simulink model "LQR_simulink_Sily_2024a"  (R2024a)
settings: Solver=FixedStepAuto  StartTime=0.0  StopTime=30  FixedStep=0.05  RelTol=1e-3
values from neighbouring files (symbols this model uses):
  Ac = LinSystem.Ac    [LQR_matlab_client_Otacky.m]    (also in LQR_matlab_client_Sily.m; LQR_sync_matlab_client.m; sync_matlab_client.m)
  b_moment = 5.4e-6    (= 5.4e-06)    [LQR_matlab_client_Otacky.m]    (also in LQR_matlab_client_Sily.m; LQR_sync_matlab_client.m; sync_matlab_client.m)
  Bc = LinSystem.Bc    [LQR_matlab_client_Otacky.m]    (also in LQR_matlab_client_Sily.m; LQR_sync_matlab_client.m; sync_matlab_client.m)
  Cc = LinSystem.Cc    [LQR_matlab_client_Otacky.m]    (also in LQR_matlab_client_Sily.m; LQR_sync_matlab_client.m; sync_matlab_client.m)
  Dc = LinSystem.Dc    [LQR_matlab_client_Otacky.m]    (also in LQR_matlab_client_Sily.m; LQR_sync_matlab_client.m; sync_matlab_client.m)
  k_thrust = 2.3e-3    (= 0.0023)    [LQR_matlab_client_Otacky.m]    (also in LQR_matlab_client_Sily.m; LQR_sync_matlab_client.m; sync_matlab_client.m)
  ki_lqr = K_ex_lqr(:, 17:20)    [LQR_koeficienty.m]
  kp_lqr = K_ex_lqr(:, 1:16)    [LQR_koeficienty.m]
  l = 0.2051    [LQR_matlab_client_Otacky.m]    (also in LQR_matlab_client_Sily.m; LQR_sync_matlab_client.m; sync_matlab_client.m)
  Q = 1e-3    (= 0.001)    [LQR_matlab_client_Otacky.m]    (also in LQR_matlab_client_Sily.m; LQR_sync_matlab_client.m; sync_matlab_client.m)
  R = 1e-4    (= 0.0001)    [LQR_matlab_client_Otacky.m]    (also in LQR_matlab_client_Sily.m; LQR_sync_matlab_client.m; sync_matlab_client.m)
  timestep = timeData.TimeStep    [LQR_matlab_client_Otacky.m]    (also in LQR_matlab_client_Sily.m; LQR_sync_matlab_client.m; sync_matlab_client.m)
  Us_p = [(M+m)*g; 0; 0; 0]    [LQR_matlab_client_Sily.m]    (also in LQR_sync_matlab_client.m)
  Xs_p = [0;0;0; 0;0;0; 0;0; 0;0;0; 0;0;0; 0;0]    [LQR_matlab_client_Otacky.m]    (also in LQR_matlab_client_Sily.m; LQR_sync_matlab_client.m)
undefined symbols (not defined in the file or in its folder): Continuous, Time
libraries: simulink_extras x5, simulink x1, ctrlSharedLib x1
settings Model: Creator=yaozhong.zhang  LastModifiedBy=Admin
settings DebuggingCC: UnconnectedInputMsg=warning  UnconnectedOutputMsg=warning  UnconnectedLineMsg=warning
settings ModelReferenceCC: EnableRefExpFcnMdlSchedulingChecks=on
settings RTWCC: GPUComputeCapability=3.5

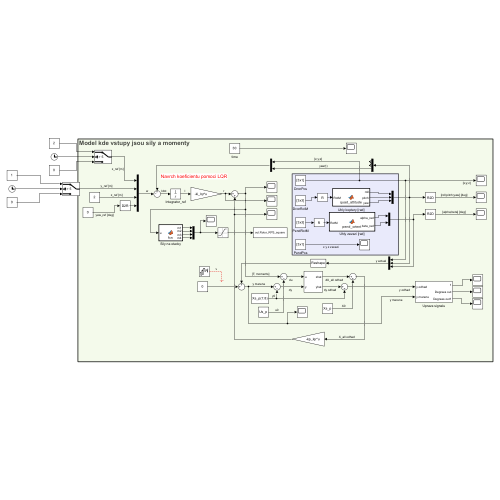
[thumbnail: Simulink's stored preview of the top-level diagram]
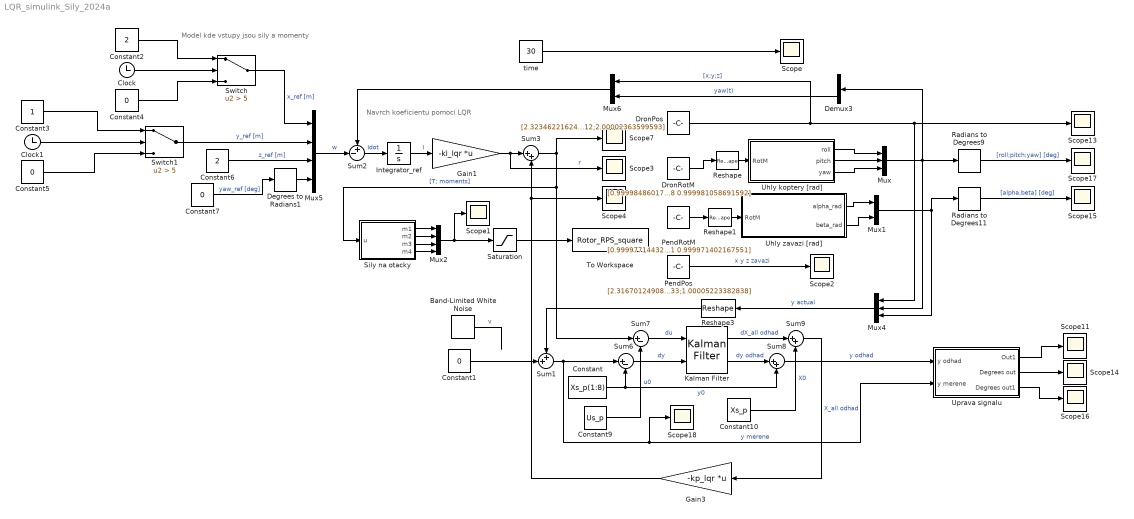
== system LQR_simulink_Sily_2024a ==
  note: Model kde vstupy jsou sily a momenty
  note: Navrch koeficientu pomoci LQR
  Band-Limited White Noise : simulink/Sources/Band-Limited White Noise  Cov=R*str2num(timestep)  Ts=str2num(timestep)  seed=[23341]
  Clock : Clock
  Clock1 : Clock
  Constant : Constant  Value=Xs_p(1:8)
  Constant{1,4..5,7} (4 alike) : Constant  Value=0
  Constant10 : Constant  Value=Xs_p
  Constant2 : Constant  Value=2
  Constant3 : Constant
  Constant6 : Constant  Value=2
  Constant9 : Constant  Value=Us_p
  Degrees to Radians1 : simulink_extras/Transformations/Degrees to Radians
  Demux3 : Demux  Outputs=3
  DronPos : Constant  Value=[2.32346221624764;1.16170882076612;2.00002363599593]  SampleTime=-1
  DronRotM : Constant  Value=[0.999984860177813 -5.50289297469162e-05 0.00550239829327193;3.98544005691727e-05 0.999996196263047 0.00275787437439109;-0.00550252912647141 -0.00275761332587778 0.999981058691592]  SampleTime=-1
  Gain1 : Gain  Gain=-ki_lqr  Multiplication=Matrix(K*u)
  Gain3 : Gain  Gain=-kp_lqr  Multiplication=Matrix(K*u)
  Integrator_ref : Integrator  InitialCondition=[1.74013379756829e-14;-1.44199272323054e-13;-17.1813439246218;-1.04137858173955e-14]
  Kalman Filter : ctrlSharedLib/Kalman Filter  TimeDomain=Continuous-Time  UseCurrentEstimator=on  ModelSource=Individual A, B, C, D matrices  ModelSourceVariable=ss(0.95,1,1,0,1)  A=Ac  B=Bc  C=Cc  D=Dc  NumberOfStates=1  NumberOfInputs=1  NumberOfOutputs=1  InitialEstimateSource=Dialog  X0=[0;0;2; 0;0;0; 0;0; 0;0;0; 0;0;0; 0;0]  P0=10  UseK=off  UseGH=off  NumberOfProcessNoiseInputs=1  G=1  TimeInvariantG=on  H=0  TimeInvariantH=on  Q=diag(Q*ones(16,1))  TimeInvariantQ=on  R=diag(R*ones(8,1))  TimeInvariantR=on  N=0  TimeInvariantN=on  AddInputPort=on  AddEnablePort=off  OutputEstimatedY=on  OutputP=off  Ts=-1
  Mux : Mux  Inputs=3
  Mux1 : Mux  Inputs=2
  Mux2 : Mux
  Mux4 : Mux  Inputs=3
  Mux5 : Mux
  Mux6 : Mux  Inputs=2
  PendPos : Constant  Value=[2.31670124908824;1.15831999056533;1.00005223382838]  SampleTime=-1
  PendRotM : Constant  Value=[0.999977144321402 -1.25651106658396e-05 0.00676096715939648;-1.03469676683034e-05 0.999994257844918 0.0033888302007973;-0.00676097091790106 -0.00338882270229201 0.999971402167551]  SampleTime=-1
  Radians to Degrees11 : simulink_extras/Transformations/Radians to Degrees
  Radians to Degrees9 : simulink_extras/Transformations/Radians to Degrees
  Reshape : Reshape  OutputDimensionality=Customize  OutputDimensions=[3,3]
  Reshape1 : Reshape  OutputDimensionality=Customize  OutputDimensions=[3,3]
  Reshape3 : Reshape  OutputDimensionality=Customize  OutputDimensions=[8,1]
  Saturation : Saturate  UpperLimit=4200  LowerLimit=0
  Scope{,1..4,7,11,13..18} (13 alike) : Scope
  Sily na otacky : MATLAB Function  TreatAsAtomicUnit=on
  Sum1 : Sum  Inputs=++|
  Sum2 : Sum  Inputs=+-|
  Sum3 : Sum  Inputs=|++
  Sum6 : Sum  Inputs=|+-
  Sum7 : Sum  Inputs=|+-
  Sum8 : Sum  Inputs=|++
  Sum9 : Sum  Inputs=|++
  Switch : Switch  Criteria=u2 > Threshold  Threshold=5  SaturateOnIntegerOverflow=off  InputSameDT=off
  Switch1 : Switch  Criteria=u2 > Threshold  Threshold=5  SaturateOnIntegerOverflow=off  InputSameDT=off
  To Workspace : ToWorkspace  VariableName=Rotor_RPS_square  SampleTime=-1
  Uhly koptery [rad] : MATLAB Function  TreatAsAtomicUnit=on
  Uhly zavazi [rad] : MATLAB Function  TreatAsAtomicUnit=on
  Uprava signalu : Subsystem
  time : Constant  Value=30  SampleTime=-1
  wires:
  DronRotM/1 -> Reshape/1
  Uhly koptery [rad]/2(pitch) -> Mux/2
  Uhly koptery [rad]/1(roll) -> Mux/1
  Uhly koptery [rad]/3(yaw) -> Mux/3
  PendPos/1 -> Scope2/1  "x y z zavazi"
  Reshape/1 -> Uhly koptery [rad]/1(RotM)
  PendRotM/1 -> Reshape1/1
  Reshape1/1 -> Uhly zavazi [rad]/1(RotM)
  Uhly zavazi [rad]/1(alpha_rad) -> Mux1/1
  Uhly zavazi [rad]/2(beta_rad) -> Mux1/2
  time/1 -> Scope/1
  Mux6/1 -> Sum2/1
  Gain3/1 -> Scope4/1, Sum3/2
  Sum2/1 -> Integrator_ref/1  "Idot"
  Switch1/1 -> Mux5/2  "y_ref [m]"
  Constant6/1 -> Mux5/3  "z_ref [m]"
  Uprava signalu/1(Out1) -> Scope11/1
  Radians to Degrees11/1 -> Scope15/1  "[alpha;beta] [deg]"
  Mux/1 -> Demux3/1, Radians to Degrees9/1, Mux4/2
  Mux4/1 -> Reshape3/1  "y actual"
  Uprava signalu/3(Degrees out1) -> Scope16/1
  Switch/1 -> Mux5/1  "x_ref [m]"
  Integrator_ref/1 -> Gain1/1  "I"
  Demux3/3 -> Mux6/2  "yaw(t)"
  Uprava signalu/2(Degrees out) -> Scope14/1
  Degrees to Radians1/1 -> Mux5/4
  Constant7/1 -> Degrees to Radians1/1  "yaw_ref [deg]"
  DronPos/1 -> Scope13/1, Mux4/1, Mux6/1  "[x;y;z]"
  Mux5/1 -> Sum2/2  "w"
  Mux1/1 -> Mux4/3, Radians to Degrees11/1
  Radians to Degrees9/1 -> Scope17/1  "[roll;pitch;yaw] [deg]"
  Sum3/1 -> Sum7/1, Sily na otacky/1(u), Scope7/1  "[T; moments]"
  Constant/1 -> Sum8/2, Sum6/2  "y0"
  Sum6/1 -> Kalman Filter/2  "dy"
  Sum9/1 -> Gain3/1  "X_all odhad"
  Band-Limited White Noise/1 -> ?  "v"
  Reshape3/1 -> Sum1/1
  Kalman Filter/1 -> Sum9/1  "dX_all odhad"
  Sum7/1 -> Kalman Filter/1  "du"
  Sum8/1 -> Uprava signalu/1(y odhad)  "y odhad"
  Constant10/1 -> Sum9/2  "X0"
  Kalman Filter/2 -> Sum8/1  "dy odhad"
  Constant9/1 -> Sum7/2  "u0"
  Sum1/1 -> Sum6/1, Uprava signalu/2(y merene), Scope18/1  "y merene"
  Gain1/1 -> Scope3/1, Sum3/1  "r"
  Constant1/1 -> Sum1/2
  Sily na otacky/2(m2) -> Mux2/2
  Sily na otacky/3(m3) -> Mux2/3
  Sily na otacky/4(m4) -> Mux2/4
  Sily na otacky/1(m1) -> Mux2/1
  Mux2/1 -> Scope1/1, Saturation/1
  Clock/1 -> Switch/2
  Constant4/1 -> Switch/3
  Constant2/1 -> Switch/1
  Constant3/1 -> Switch1/1
  Clock1/1 -> Switch1/2
  Constant5/1 -> Switch1/3
  Saturation/1 -> To Workspace/1

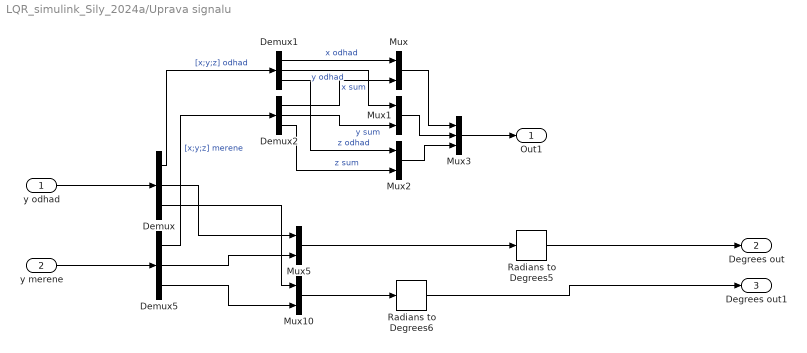
== system LQR_simulink_Sily_2024a/Uprava signalu ==
  y odhad : Inport
  y merene : Inport  Port=2
  Demux{,1..2,5} (4 alike) : Demux  Outputs=3
  Mux{,1..2,5,10} (5 alike) : Mux  Inputs=2
  Mux3 : Mux  Inputs=3
  Radians to Degrees5 : simulink_extras/Transformations/Radians to Degrees
  Radians to Degrees6 : simulink_extras/Transformations/Radians to Degrees
  Out1 : Outport
  Degrees out : Outport  Port=2
  Degrees out1 : Outport  Port=3
  wires:
  Demux5/3 -> Mux10/2
  Demux/3 -> Mux10/1
  Mux5/1 -> Radians to Degrees5/1
  Demux/2 -> Mux5/1
  Demux5/2 -> Mux5/2
  Demux5/1 -> Demux2/1  "[x;y;z] merene"
  Demux/1 -> Demux1/1  "[x;y;z] odhad"
  Mux10/1 -> Radians to Degrees6/1
  y odhad/1 -> Demux/1
  Radians to Degrees6/1 -> Degrees out1/1
  Radians to Degrees5/1 -> Degrees out/1
  y merene/1 -> Demux5/1
  Demux1/1 -> Mux/1  "x odhad"
  Demux2/1 -> Mux/2  "x sum"
  Demux1/2 -> Mux1/1  "y odhad"
  Demux2/2 -> Mux1/2  "y sum"
  Mux/1 -> Mux3/1
  Mux1/1 -> Mux3/2
  Mux2/1 -> Mux3/3
  Demux1/3 -> Mux2/1  "z odhad"
  Demux2/3 -> Mux2/2  "z sum"
  Mux3/1 -> Out1/1

== matlab function LQR_simulink_Sily_2024a/Uhly zavazi [rad] ==
  data: RotM input; alpha_rad output; beta_rad output
function [alpha_rad, beta_rad] = pend_orient(RotM)
% Расчет углов альфа и бета маятника

% Вектор маятника
rope_vector = RotM * [0; 0; -1];

% Расчет угла альфа
rope_vector_xz = rope_vector([1, 3]); % Компоненты x и z
z_axis = [0; -1];
cos_alpha = dot(rope_vector_xz, z_axis) / (norm(rope_vector_xz) * norm(z_axis));
cos_alpha = max(-1, min(1, cos_alpha)); % Ограничиваем в диапазоне [-1, 1]
alpha = acos(cos_alpha);
if rope_vector(1) < 0
    alpha = -alpha;
end

% Расчет угла бета
rope_vector_xz_3 = [rope_vector(1); 0; rope_vector(3)];
cos_beta = dot(rope_vector, rope_vector_xz_3) / (norm(rope_vector) * norm(rope_vector_xz_3));
cos_beta = max(-1, min(1, cos_beta)); % Ограничиваем в диапазоне [-1, 1]
beta = acos(cos_beta);
if rope_vector(2) < 0
    beta = -beta;
end

% Округляем до 5 знаков после запятой
% alpha_rad = round(alpha, 5); %[rad]
% beta_rad = round(beta, 5); %[rad]
alpha_rad = alpha;
beta_rad = beta;

== matlab function LQR_simulink_Sily_2024a/Sily na otacky ==
  data: u input; m1 output; m2 output; m3 output; m4 output; b_moment parameter; k_thrust parameter; l parameter
function [m1, m2, m3, m4]= fcn(u, b_moment, k_thrust, l)

T = u(1);
Tau_phi = u(2);
Tau_theta = u(3);
Tau_psi = u(4);

m1 = ( (Tau_phi*b_moment - Tau_theta*b_moment + l*T*b_moment + l*Tau_psi*k_thrust)/(4*l*b_moment*k_thrust));
m2 = ( (-Tau_theta*b_moment - Tau_phi*b_moment + l*T*b_moment - l*Tau_psi*k_thrust)/(4*l*b_moment*k_thrust));
m3 = ( (Tau_theta*b_moment - Tau_phi*b_moment + l*T*b_moment + l*Tau_psi*k_thrust)/(4*l*b_moment*k_thrust));
m4 = ( (Tau_phi*b_moment + Tau_theta*b_moment + l*T*b_moment - l*Tau_psi*k_thrust)/(4*l*b_moment*k_thrust));

== matlab function LQR_simulink_Sily_2024a/Uhly koptery [rad] ==
  data: RotM input; roll output; pitch output; yaw output
function [roll, pitch, yaw] = quad_attitude(RotM)
% matice rotace koptery z Python, vuci svetu!!!
% rotm2eul prevadi na Eulerove uhly
radians = rotm2eul(RotM, 'ZYX'); % pouzivam poradi ZYX

% roll = kolem x, pitch = kolem y, yaw = kolem z
yaw = radians(1);
pitch = radians(2);
roll = radians(3);
end
